simulink model "DCMotorLoopwBacklash"  (R2015a)
settings: Solver=ode45  StartTime=0.0  StopTime=35  RelTol=1e-8  AbsTol=1e-8
values from neighbouring files (symbols this model uses):
  c = 0.001    [CSD_HW_1_Script.m]    (also in Plotshit.m)
  d = 5*pi/180    (= 0.0872664625997)    [CSD_HW_1_Script.m]    (also in Plotshit.m)
  Jl = 0.02    [CSD_HW_1_Script.m]    (also in Plotshit.m)
  Jm = 0.001    [CSD_HW_1_Script.m]    (also in Plotshit.m)
  K = [0.1 30]    [CSD_HW_1_Script.m]    (also in Plotshit.m)
  Kt = 0.03    [CSD_HW_1_Script.m]    (also in Plotshit.m)
  L = 0    [CSD_HW_1_Script.m]    (also in Plotshit.m = C*P)
  N = 3    [CSD_HW_1_Script.m]    (also in Plotshit.m)
  R = 0.1    [CSD_HW_1_Script.m]    (also in Plotshit.m)
settings Model: Creator=yarde_000  LastModifiedBy=yarde_000

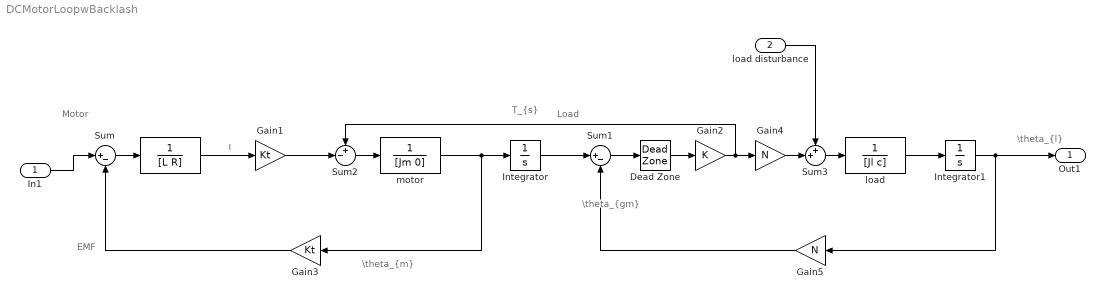
== system DCMotorLoopwBacklash ==
  note: Load
  note: Motor
  note: \theta_{m}
  note: EMF
  note: T_{s}
  note: \theta_{l}
  note: \theta_{gm}
  In1 : Inport
  load disturbance : Inport  Port=2
  " " : TransferFcn  Denominator=[L R]
  " load" : TransferFcn  Denominator=[Jl c]
  " motor" : TransferFcn  Denominator=[Jm 0]
  Dead Zone : DeadZone  LowerValue=-d/2  UpperValue=d/2  SaturateOnIntegerOverflow=on
  Gain1 : Gain  Gain=Kt
      mask Display: disp('K_t','texmode','on')
  Gain2 : Gain  Gain=K
      mask Display: disp('K','texmode','on')
  Gain3 : Gain  Gain=Kt
      mask Display: disp('K_t','texmode','on')
  Gain4 : Gain  Gain=N
      mask Display: disp('N','texmode','on')
  Gain5 : Gain  Gain=N
      mask Display: disp('N','texmode','on')
  Integrator : Integrator
  Integrator1 : Integrator
  Sum : Sum  Inputs=|+-
  Sum1 : Sum  Inputs=|+-
  Sum2 : Sum  Inputs=+-|
  Sum3 : Sum  Inputs=++|
  Out1 : Outport
  wires:
  Sum/1 -> " "/1
  " "/1 -> Gain1/1  "I"
  " motor"/1 -> Gain3/1, Integrator/1
  Gain3/1 -> Sum/2
  Integrator/1 -> Sum1/1
  Sum1/1 -> Dead Zone/1
  Dead Zone/1 -> Gain2/1
  Gain1/1 -> Sum2/2
  Sum2/1 -> " motor"/1
  " load"/1 -> Integrator1/1
  Integrator1/1 -> Out1/1, Gain5/1
  Gain5/1 -> Sum1/2
  In1/1 -> Sum/1
  Gain4/1 -> Sum3/2
  Sum3/1 -> " load"/1
  load disturbance/1 -> Sum3/1
  Gain2/1 -> Sum2/1, Gain4/1
